simulink model "dc_dc_hb"  (Simulink 6.1)
settings: Solver=ode23tb  StartTime=0.0  StopTime=0.001  MaxStep=1e-7  RelTol=1e-3  AbsTol=.01
libraries: powerlib x12
settings Model: LastModifiedBy=ThinkPad
settings DebuggingCC: SolverPrmCheckMsg=warning

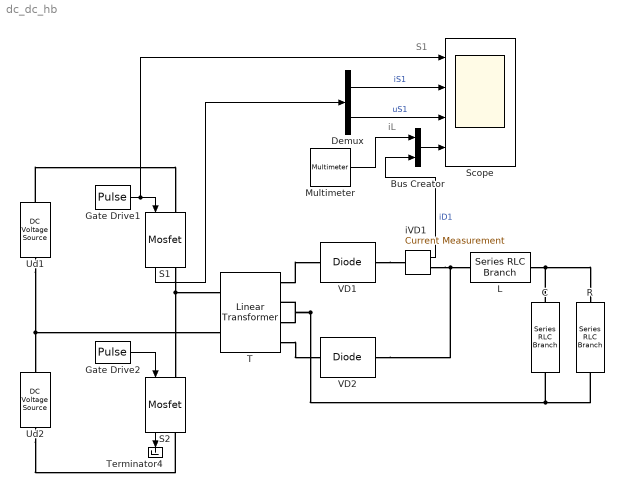
== system dc_dc_hb ==
  note: S1
  note: iL
  Bus Creator : BusCreator  DialogController=Simulink.DDGSource_Bus  Inputs=2
  C : powerlib/Elements/Series RLC Branch  Orientation=up  PhysicalDomain=powersysdomain  SubClassName=unknown  LeftPortType=p1  RightPortType=p1  LConnTagsString=__new0  RConnTagsString=__new0  Resistance=0  Inductance=0  Capacitance=2e-5  Measurements=None
  Demux : Demux  Outputs=2
  Gate Drive1 : DiscretePulseGenerator  PulseType=Time based  Period=0.00005  PulseWidth=30
  Gate Drive2 : DiscretePulseGenerator  PulseType=Time based  Period=0.00005  PulseWidth=30  PhaseDelay=0.000025
  L : powerlib/Elements/Series RLC Branch  PhysicalDomain=powersysdomain  SubClassName=unknown  LeftPortType=p1  RightPortType=p1  LConnTagsString=__new0  RConnTagsString=__new0  Resistance=0  Inductance=1e-4  Capacitance=inf  Measurements=Branch voltage and current
  Multimeter : powerlib/Measurements/Multimeter  PhasorSimulation=off  OutputType=Complex  sel=6  L=6  Gain=1  yselected={'Ib: L'};  PSBOutputType=1  PSBequivalent=0  AxesSetting=[0,0.1,-100,100]  Display=0  SavedBlockNames=-11
  R : powerlib/Elements/Series RLC Branch  Orientation=down  PhysicalDomain=powersysdomain  SubClassName=unknown  LeftPortType=p1  RightPortType=p1  LConnTagsString=__new0  RConnTagsString=__new0  Resistance=2  Inductance=0  Capacitance=inf  Measurements=Branch voltage
  S1 : powerlib/Power Electronics/Mosfet  Orientation=down  Ron=0.01  Lon=1e-8  Rd=.01  IC=0  Rs=30  Cs=1e-8  Measurements=on
  S2 : powerlib/Power Electronics/Mosfet  Orientation=down  Ron=0.01  Lon=1e-8  Rd=.01  IC=0  Rs=30  Cs=1e-8  Measurements=on
  Scope : Scope  NumInputPorts=4
      settings: TimeRange=0.0005  YMin=0~-5~0~-5  YMax=2~25~250~20  SampleTime=1e-7
  T : powerlib/Elements/Linear Transformer  PhysicalDomain=powersysdomain  SubClassName=unknown  LeftPortType=p1  RightPortType=p1  LConnTagsString=a|b  RConnTagsString=A|B|C|D  NominalPower=[1000 20000 ]  winding1="[ 100  0.002  0.002 ]"  winding2="[ 50  0.002  0.002 ]"  ThreeWindings=on  winding3=[ 50 0.002 0.002 ]  RmLm=[ 500 20 ]  Measurements=Winding voltages
  Terminator4 : Terminator
      settings: Orientation=down
  Ud1 : powerlib/Electrical Sources/DC Voltage Source  Orientation=up  Amplitude=100  Measurements=None
  Ud2 : powerlib/Electrical Sources/DC Voltage Source  Orientation=up  Amplitude=100  Measurements=None
  VD1 : powerlib/Power Electronics/Diode  Ron=0.001  Lon=0  Vf=0.8  IC=0  Rs=100  Cs=1e-9  Measurements=off
  VD2 : powerlib/Power Electronics/Diode  Ron=0.001  Lon=0  Vf=0.8  IC=0  Rs=100  Cs=1e-9  Measurements=off
  iVD1 : powerlib/Measurements/Current Measurement  PhasorSimulation=off  OutputType=Complex  PSBequivalent=0
  wires:
  Gate Drive2/1 -> S2/1
  Gate Drive1/1 -> S1/1, Scope/1
  Multimeter/1 -> Bus Creator/1
  iVD1/1 -> Bus Creator/2  "iD1"
  S2/1 -> Terminator4/1
  S1/1 -> Demux/1
  Demux/1 -> Scope/2  "iS1"
  Demux/2 -> Scope/3  "uS1"
  Bus Creator/1 -> Scope/4
  connections:
  Ud2/LConn1 -- S2/RConn1
  S1/RConn1 -- S2/LConn1 -- T/LConn1
  Ud1/RConn1 -- S1/LConn1
  Ud1/LConn1 -- Ud2/RConn1 -- T/LConn2
  T/RConn3 -- T/RConn2 -- R/RConn1 -- C/LConn1
  T/RConn1 -- VD1/LConn1
  T/RConn4 -- VD2/LConn1
  VD2/RConn1 -- L/LConn1 -- iVD1/RConn1
  L/RConn1 -- R/LConn1 -- C/RConn1
  VD1/RConn1 -- iVD1/LConn1
